simulink model "untitled3"  (R2025a)
settings: Solver=VariableStepAuto  StartTime=0.0  StopTime=10.0  RelTol=1e-3
settings Model: Creator=Win 11  LastModifiedBy=Win 11

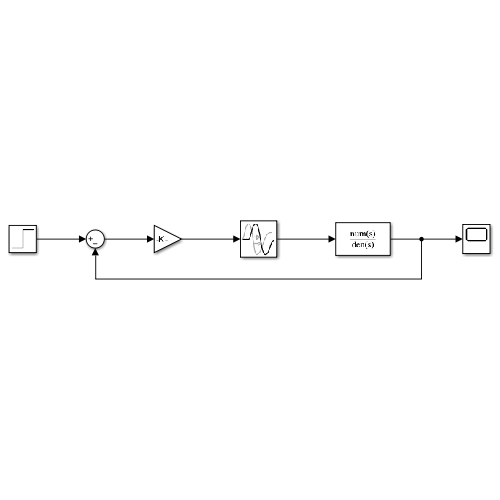
[thumbnail: Simulink's stored preview of the top-level diagram]
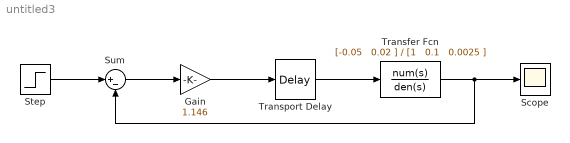
== system untitled3 ==
  Gain : Gain  Gain=1.146
  Scope : Scope
      settings: ActiveDisplayYMinimum=-0.40302339213455979  ActiveDisplayYMaximum=0.33424140788910567
  Step : Step  Before=-4  After=4  SampleTime=0
  Sum : Sum  Inputs=|+-
  Transfer Fcn : TransferFcn  Numerator=|  Denominator=|
      Numerator=|
      | [-0.05   0.02
      | ]
      Denominator=|
      | [1   0.1   0.0025
      | ]
  Transport Delay : TransportDelay  DelayTime=2
  wires:
  Step/1 -> Sum/1
  Sum/1 -> Gain/1
  Gain/1 -> Transport Delay/1
  Transport Delay/1 -> Transfer Fcn/1
  Transfer Fcn/1 -> Sum/2, Scope/1
